simulink model "Tutorial24"  (R2020a)
settings: Solver=FixedStepDiscrete  StartTime=0.0  StopTime=10.0  FixedStep=1  RelTol=1e-3
values from neighbouring files (symbols this model uses):
  InitSeq = [0 0 0 0 0 0]    [matlab.mat]
libraries: simulink x2
settings Model: Creator=ashok  LastModifiedBy=ashok

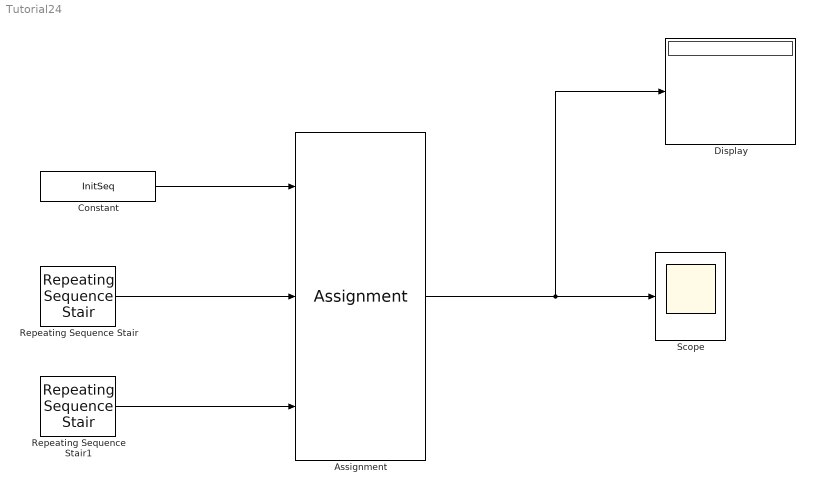
== system Tutorial24 ==
  Assignment : Assignment  IndexMode=Zero-based  DiagnosticForDimensions=Warning  IndexOptions=Index vector (port)  Indices=1  OutputSizes=1
  Constant : Constant  Value=InitSeq
  Display : Display
  Repeating Sequence Stair : simulink/Sources/Repeating Sequence Stair  OutValues=[3 1 4 2 1].'  tsamp=-1  OutMin=[]  OutMax=[]  OutDataTypeStr=double  OutputDataTypeScalingMode=double  OutDataType=fixdt(0,8)  ConRadixGroup=Best Precision: Vector-wise  OutScaling=2^-12
  Repeating Sequence Stair1 : simulink/Sources/Repeating Sequence Stair  OutValues=Index_Vector_Rev  tsamp=-1  OutMin=[]  OutMax=[]  OutDataTypeStr=double  OutputDataTypeScalingMode=double  OutDataType=fixdt(0,8)  ConRadixGroup=Best Precision: Vector-wise  OutScaling=2^-12
  Scope : Scope
  wires:
  Constant/1 -> Assignment/1
  Repeating Sequence Stair/1 -> Assignment/2
  Repeating Sequence Stair1/1 -> Assignment/3
  Assignment/1 -> Display/1, Scope/1
